simulink model "TC_track"  (R2026a)
settings: Solver=FixedStepDiscrete  StopTime=timeMax  FixedStep=Ts_plant
InitFcn:
  | TC_paramsOnly = true;
  | run('params_track.m');
  | clear TC_paramsOnly
values from neighbouring files (symbols this model uses):
  aeroFrontFraction = 0.50    (= 0.5)    [TC_parameters.m]    (also in params.m; params_track.m)
  CDA = 1.20    (= 1.2)    [TC_parameters.m]    (also in params.m; params_track.m)
  cg_f = W * rearWeightFraction    (= 0.765175)    [TC_parameters.m]    (also in params.m; params_track.m)
  cg_r = W * frontWeightFraction    (= 0.765175)    [TC_parameters.m]    (also in params.m; params_track.m)
  CLA = 4.40    (= 4.4)    [TC_parameters.m]    (also in params.m; params_track.m)
  Cmax = 0    [TC_parameters.m]    (also in params.m = 5.375; params_track.m = 5.375)
  Cmin = -Max_Motor_Torque    (= -21.5)    [TC_parameters.m]    (also in params.m; params_track.m)
  Course_Length = Track_Length    [params_track.m]
  Drive_Train = 0.85    [TC_parameters.m]    (also in params.m = 0.92; params_track.m = 0.92)
  Driver_Brake_Band = 1.0    (= 1)    [params_track.m]
  Driver_Brake_Max_Decel = 1.5*gravity    (= 14.709975)    [params_track.m]
  Driver_Lift_Band = 0.5    [params_track.m]
  Driver_Line_Recovery_Hz = 0.3    [params_track.m]
  Driver_Preview_Time = 0.3    [params_track.m]
  Driver_Speed_Target = speedCap*ones(size(Track_Curvature))    [params_track.m]
  fd = 12.5    [TC_parameters.m]    (also in params.m; params_track.m)
  Feedforward_FallRate_FL = 2000    [params.m]    (also in params_track.m)
  Feedforward_FallRate_FR = 2000    [params.m]    (also in params_track.m)
  Feedforward_FallRate_RL = 2000    [params.m]    (also in params_track.m)
  Feedforward_FallRate_RR = 2000    [params.m]    (also in params_track.m)
  Feedforward_Filter_Alpha = 1 - exp(-2*pi*Feedforward_Filter_Hz*Ts)    [params.m]    (also in params_track.m)
  Feedforward_InitialState_FL = muFz_front_launch / Feedforward_Filter_Alpha    [params.m]    (also in params_track.m)
  Feedforward_InitialState_FR = Feedforward_InitialState_FL    [params.m]    (also in params_track.m)
  Feedforward_InitialState_RL = muFz_rear_launch / Feedforward_Filter_Alpha    [params.m]    (also in params_track.m)
  Feedforward_InitialState_RR = Feedforward_InitialState_RL    [params.m]    (also in params_track.m)
  Feedforward_Launch_FL = min(Max_Motor_Torque, Kff_FL*r/(fd*Drive_Train) *      muFz_front_launch*targetForceShape(Slip_Target_FL))    [params.m]    (also in params_track.m)
  Feedforward_Launch_FR = min(Max_Motor_Torque, Kff_FR*r/(fd*Drive_Train) *      muFz_front_launch*targetForceShape(Slip_Target_FR))    [params.m]    (also in params_track.m)
  Feedforward_Launch_RL = min(Max_Motor_Torque, Kff_RL*r/(fd*Drive_Train) *      muFz_rear_launch*targetForceShape(Slip_Target_RL))    [params.m]    (also in params_track.m)
  Feedforward_Launch_RR = min(Max_Motor_Torque, Kff_RR*r/(fd*Drive_Train) *      muFz_rear_launch*targetForceShape(Slip_Target_RR))    [params.m]    (also in params_track.m)
  Feedforward_RiseRate_FL = 800    [params.m]    (also in params_track.m)
  Feedforward_RiseRate_FR = 800    [params.m]    (also in params_track.m)
  Feedforward_RiseRate_RL = 800    [params.m]    (also in params_track.m)
  Feedforward_RiseRate_RR = 800    [params.m]    (also in params_track.m)
  Fz_front_static = Mv * gravity * cg_r / W    (= 1387.6672151)    [TC_parameters.m]    (also in params.m; params_track.m)
  Fz_rear_static = Mv * gravity * cg_f / W    (= 1387.6672151)    [TC_parameters.m]    (also in params.m; params_track.m)
  Grip_Fact = 1.0    (= 1)    [TC_parameters.m]    (also in params.m = 0.6; params_track.m = 0.6)
  h_cg = 10.4 * in_to_m    (= 0.26416)    [TC_parameters.m]    (also in params.m; params_track.m)
  J_wheel_side = 0.45    [TC_parameters.m]    (also in params.m = 0.35; params_track.m = 0.35)
  Kaw_FL = Ki_FL / Kp_FL    (= 32)    [params.m]    (also in params_track.m)
  Kaw_FR = Ki_FR / Kp_FR    (= 32)    [params.m]    (also in params_track.m)
  Kaw_RL = Ki_RL / Kp_RL    (= 12)    [params.m]    (also in params_track.m)
  Kaw_RR = Ki_RR / Kp_RR    (= 12)    [params.m]    (also in params_track.m)
  Kd_FL = 0    [TC_parameters.m]    (also in params.m; params_track.m)
  Kd_FR = 0    [TC_parameters.m]    (also in params.m; params_track.m)
  Kd_RL = 0    [TC_parameters.m]    (also in params.m; params_track.m)
  Kd_RR = 0    [TC_parameters.m]    (also in params.m; params_track.m)
  Kff_FL = 0.9    [params.m]    (also in params_track.m)
  Kff_FR = 0.9    [params.m]    (also in params_track.m)
  Kff_RL = 0.9    [params.m]    (also in params_track.m)
  Kff_RR = 0.9    [params.m]    (also in params_track.m)
  Ki_FL = 180    [TC_parameters.m]    (also in params.m = 480; params_track.m = 480)
  Ki_FR = 180    [TC_parameters.m]    (also in params.m = 480; params_track.m = 480)
  Ki_RL = 180    [TC_parameters.m]    (also in params.m = 240; params_track.m = 240)
  Ki_RR = 180    [TC_parameters.m]    (also in params.m = 240; params_track.m = 240)
  Kp_FL = 32    [TC_parameters.m]    (also in params.m = 15; params_track.m = 15)
  Kp_FR = 32    [TC_parameters.m]    (also in params.m = 15; params_track.m = 15)
  Kp_RL = 32    [TC_parameters.m]    (also in params.m = 20; params_track.m = 20)
  Kp_RR = 32    [TC_parameters.m]    (also in params.m = 20; params_track.m = 20)
  Ktrack_FL = 50    [params.m]    (also in params_track.m)
  Ktrack_FR = 50    [params.m]    (also in params_track.m)
  Ktrack_RL = 50    [params.m]    (also in params_track.m)
  Ktrack_RR = 50    [params.m]    (also in params_track.m)
  Lateral_Mu_Ratio = 1.00    (= 1)    [params_track.m]
  Launch_Pedal_Initial = T_request_per_motor    (= 21.5)    [params.m]    (also in params_track.m)
  LLTD_Front = 0.50    (= 0.5)    [params_track.m]
  Max_Motor_Torque = 21.5    [TC_parameters.m]    (also in params.m; params_track.m)
  Max_Wheel_Omega = Max_Motor_RPM * 2*pi/60 / fd    (= 167.551608191)    [TC_parameters.m]    (also in params.m; params_track.m)
  maxTractivePower = 80e3    (= 80000)    [TC_parameters.m]    (also in params.m; params_track.m)
  motorInverterEfficiency = 1.00    (= 1)    [params.m]    (also in params_track.m)
  Mv = vehicleMassNoDriver + driverMass    (= 283.00535149)    [TC_parameters.m]    (also in params.m; params_track.m)
  Pacejka_B = 10.400    (= 10.4)    [TC_parameters.m]    (also in params.m; params_track.m)
  Pacejka_C = -1.580    (= -1.58)    [TC_parameters.m]    (also in params.m; params_track.m)
  Pacejka_D1 = -3.020    (= -3.02)    [TC_parameters.m]    (also in params.m; params_track.m)
  Pacejka_D2 = 0.800    (= 0.8)    [TC_parameters.m]    (also in params.m; params_track.m)
  r = 0.5 * 16.0 * in_to_m    (= 0.2032)    [TC_parameters.m]    (also in params.m; params_track.m; slip_estimator.m = ay / vref0)
  rho = 1.225    [TC_parameters.m]    (also in params.m; params_track.m)
  Slip_Filter_Alpha = 1 - exp(-2*pi*Slip_Filter_Hz*Ts)    [params.m]    (also in params_track.m)
  Slip_Target_FL = 0.12    [TC_parameters.m]    (also in params.m; params_track.m)
  Slip_Target_FR = 0.12    [TC_parameters.m]    (also in params.m; params_track.m)
  Slip_Target_RL = 0.12    [TC_parameters.m]    (also in params.m = 0.145; params_track.m = 0.145)
  Slip_Target_RR = 0.12    [TC_parameters.m]    (also in params.m = 0.145; params_track.m = 0.145)
  slipSpeedFloor = 0.50    (= 0.5)    [TC_parameters.m]    (also in params.m; params_track.m)
  Speed_Limit_Taper_Omega = Speed_Limit_Taper_RPM * 2*pi/60 / fd    (= 4.18879020479)    [params.m]    (also in params_track.m)
  Surface_Breakpoints = unique(surfaceBreaks)    [params_track.m]
  Surface_Grip_Table = Grip_Fact*ones(2, numel(Surface_Breakpoints))    [params_track.m]
  tau_motor = 0.03    [TC_parameters.m]    (also in params.m = 0.005; params_track.m = 0.005)
  Track_Breakpoints = double(misTrack.s_m(:))    [params_track.m]
  Track_Curvature = atGpsDistance(misTrack.curvature_1pm)    [params_track.m]
  trackFront = 49.0 * in_to_m    (= 1.2446)    [TC_parameters.m]    (also in params.m; params_track.m)
  trackRear = 49.0 * in_to_m    (= 1.2446)    [TC_parameters.m]    (also in params.m; params_track.m)
  Ts = 0.002    [TC_parameters.m]    (also in params.m; params_track.m)
  Ts_plant = 0.0001    [params.m]    (also in params_track.m)
  W = 60.25 * in_to_m    (= 1.53035)    [TC_parameters.m]    (also in params.m; params_track.m)
  Wheel_Lateral_Position = [trackFront/2; -trackFront/2;      trackRear/2; -trackRear/2]    [params_track.m]
  Wheel_Longitudinal_Position = [cg_f; cg_f; -cg_r; -cg_r]    [params_track.m]
  Wheel_Side = [1; 2; 1; 2]    [params_track.m]
undefined symbols (not defined in the file or in its folder): DiscIntNeverNeededParam
libraries: slpidlib x4
(part 1 of 2)
settings Model: Creator=jacks  LastModifiedBy=jacks

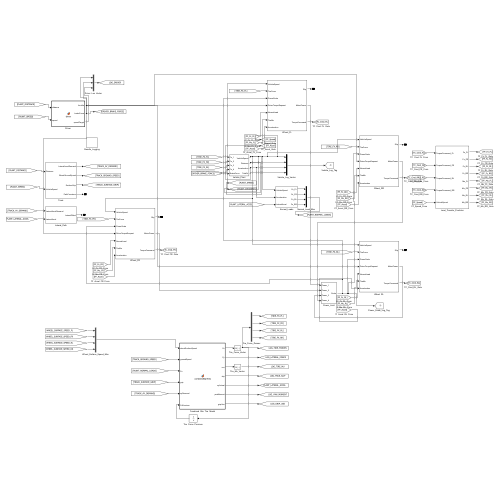
[thumbnail: Simulink's stored preview of the top-level diagram]
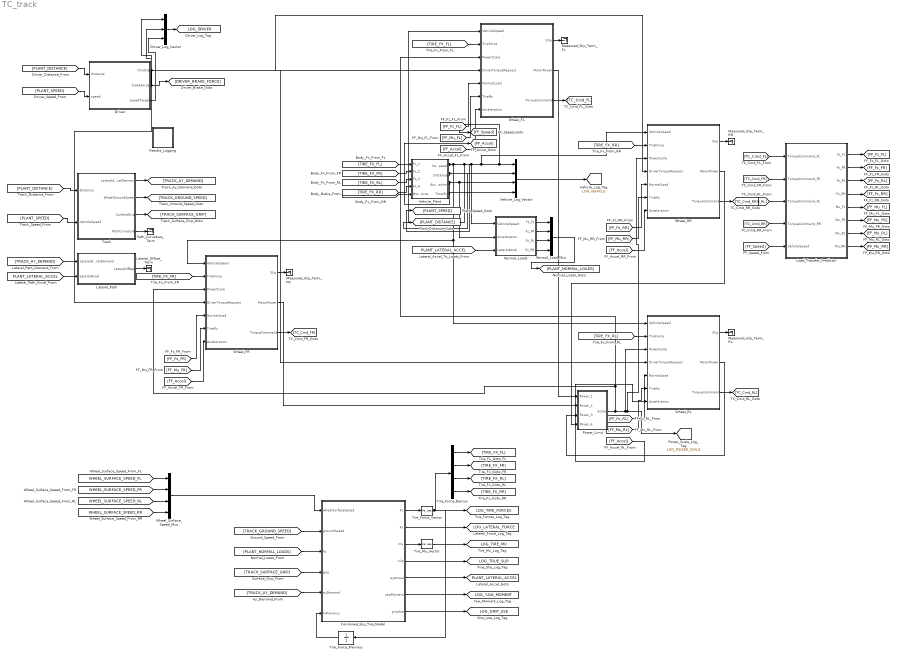
== system TC_track ==
  Combined_Slip_Tire_Model : MATLAB Function  TreatAsAtomicUnit=on
  Driver : MATLAB Function  TreatAsAtomicUnit=on
  Driver_Log_Vector : Mux  Inputs=3
  Lateral_Offset_Term : Terminator
  Lateral_Path : Subsystem  Description=Offset of the car left of the line. While the tires are short of the lateral acceleration the line needs, the car drifts by the difference; otherwise the driver steers back at Driver_Line_Recovery_Hz.
  Load_Transfer_Predictor : Subsystem
  Measured_Slip_Term_FL : Terminator
  Measured_Slip_Term_FR : Terminator
  Measured_Slip_Term_RL : Terminator
  Measured_Slip_Term_RR : Terminator
  Normal_Load_Mux : Mux
  Normal_Loads : Subsystem
  Path_Curvature_Term : Terminator
  Power_Limit : Subsystem
  Results_Logging : Subsystem
  Tire_Force_Demux : Demux
  Tire_Force_Previous : UnitDelay  InitialCondition=zeros(4,1)  SampleTime=Ts_plant
  Tire_Force_Vector : Reshape
  Tire_Mu_Vector : Reshape
  Track : Subsystem  Description=Track: path curvature, lateral-acceleration demand, per-wheel ground speeds, and per-wheel surface grip along the course.
  Vehicle_Log_Vector : Mux
  Vehicle_Plant : Subsystem
  Wheel_FL : Subsystem
  Wheel_FR : Subsystem
  Wheel_RL : Subsystem
  Wheel_RR : Subsystem
  Wheel_Surface_Speed_Mux : Mux
  tag scope: LOG_DRIVER=global, LOG_GRIP_USE=global, LOG_LATERAL_FORCE=global, LOG_POWER_SCALE=global, LOG_TIRE_FORCES=global, LOG_TIRE_MU=global, LOG_TRUE_SLIP=global, LOG_VEHICLE=global, LOG_YAW_MOMENT=global, PLANT_LATERAL_ACCEL=global
  wires:
  Power_Limit/1(Scale) -> [LOG_POWER_SCALE], Wheel_RR/3(PowerScale), Wheel_RL/3(PowerScale), Wheel_FR/3(PowerScale), Wheel_FL/3(PowerScale)
  Wheel_RR/2(MotorPower) -> Power_Limit/4(Power_4)
  Vehicle_Plant/1(VehicleSpeed) -> [FF_Speed], Vehicle_Log_Vector/1, Wheel_RR/1(VehicleSpeed), Normal_Loads/1(VehicleSpeed), Wheel_FL/1(VehicleSpeed), Wheel_RL/1(VehicleSpeed), Wheel_FR/1(VehicleSpeed), [PLANT_SPEED]
  Vehicle_Plant/3(Acceleration) -> Normal_Loads/2(Acceleration), Vehicle_Log_Vector/3, [FF_Accel]
  Vehicle_Plant/4(TotalFx) -> Vehicle_Log_Vector/4
  Vehicle_Plant/2(Distance) -> Vehicle_Log_Vector/2, [PLANT_DISTANCE]
  Wheel_RL/2(MotorPower) -> Power_Limit/3(Power_3)
  Wheel_FR/2(MotorPower) -> Power_Limit/2(Power_2)
  Wheel_FL/2(MotorPower) -> Power_Limit/1(Power_1)
  Vehicle_Log_Vector/1 -> [LOG_VEHICLE]
  [FF_Fz_FL] -> Wheel_FL/5(NormalLoad)
  [FF_Mu_FL] -> Wheel_FL/6(TireMu)
  [FF_Accel] -> Wheel_FL/7(Acceleration)
  [FF_Fz_FR] -> Wheel_FR/5(NormalLoad)
  [FF_Mu_FR] -> Wheel_FR/6(TireMu)
  [FF_Accel] -> Wheel_FR/7(Acceleration)
  [FF_Fz_RL] -> Wheel_RL/5(NormalLoad)
  [FF_Mu_RL] -> Wheel_RL/6(TireMu)
  [FF_Accel] -> Wheel_RL/7(Acceleration)
  [FF_Fz_RR] -> Wheel_RR/5(NormalLoad)
  [FF_Mu_RR] -> Wheel_RR/6(TireMu)
  [FF_Accel] -> Wheel_RR/7(Acceleration)
  Wheel_FL/3(TorqueCommand) -> [TC_Cmd_FL]
  [TC_Cmd_FL] -> Load_Transfer_Predictor/1(TorqueCommand_FL)
  Load_Transfer_Predictor/1(Fz_FL) -> [FF_Fz_FL]
  Load_Transfer_Predictor/5(Mu_FL) -> [FF_Mu_FL]
  Wheel_FR/3(TorqueCommand) -> [TC_Cmd_FR]
  [TC_Cmd_FR] -> Load_Transfer_Predictor/2(TorqueCommand_FR)
  Load_Transfer_Predictor/2(Fz_FR) -> [FF_Fz_FR]
  Load_Transfer_Predictor/6(Mu_FR) -> [FF_Mu_FR]
  Wheel_RL/3(TorqueCommand) -> [TC_Cmd_RL]
  [TC_Cmd_RL] -> Load_Transfer_Predictor/3(TorqueCommand_RL)
  Load_Transfer_Predictor/3(Fz_RL) -> [FF_Fz_RL]
  Load_Transfer_Predictor/7(Mu_RL) -> [FF_Mu_RL]
  Wheel_RR/3(TorqueCommand) -> [TC_Cmd_RR]
  [TC_Cmd_RR] -> Load_Transfer_Predictor/4(TorqueCommand_RR)
  Load_Transfer_Predictor/4(Fz_RR) -> [FF_Fz_RR]
  Load_Transfer_Predictor/8(Mu_RR) -> [FF_Mu_RR]
  [FF_Speed] -> Load_Transfer_Predictor/5(VehicleSpeed)
  Wheel_FL/1(Slip) -> Measured_Slip_Term_FL/1
  Wheel_FR/1(Slip) -> Measured_Slip_Term_FR/1
  Wheel_RL/1(Slip) -> Measured_Slip_Term_RL/1
  Wheel_RR/1(Slip) -> Measured_Slip_Term_RR/1
  [PLANT_DISTANCE] -> Track/1(Distance)
  [PLANT_SPEED] -> Track/2(VehicleSpeed)
  Track/1(LateralAccelDemand) -> [TRACK_AY_DEMAND]
  Track/2(WheelGroundSpeed) -> [TRACK_GROUND_SPEED]
  Track/3(SurfaceGrip) -> [TRACK_SURFACE_GRIP]
  Track/4(PathCurvature) -> Path_Curvature_Term/1
  Normal_Loads/1(Fz_FL) -> Normal_Load_Mux/1
  Normal_Loads/2(Fz_FR) -> Normal_Load_Mux/2
  Normal_Loads/3(Fz_RL) -> Normal_Load_Mux/3
  Normal_Loads/4(Fz_RR) -> Normal_Load_Mux/4
  Normal_Load_Mux/1 -> [PLANT_NORMAL_LOADS]
  [PLANT_LATERAL_ACCEL] -> Normal_Loads/3(LateralAccel)
  [WHEEL_SURFACE_SPEED_FL] -> Wheel_Surface_Speed_Mux/1
  [WHEEL_SURFACE_SPEED_FR] -> Wheel_Surface_Speed_Mux/2
  [WHEEL_SURFACE_SPEED_RL] -> Wheel_Surface_Speed_Mux/3
  [WHEEL_SURFACE_SPEED_RR] -> Wheel_Surface_Speed_Mux/4
  Wheel_Surface_Speed_Mux/1 -> Combined_Slip_Tire_Model/1(wheelSurfaceSpeed)
  [TRACK_GROUND_SPEED] -> Combined_Slip_Tire_Model/2(groundSpeed)
  [PLANT_NORMAL_LOADS] -> Combined_Slip_Tire_Model/3(Fz)
  [TRACK_SURFACE_GRIP] -> Combined_Slip_Tire_Model/4(grip)
  [TRACK_AY_DEMAND] -> Combined_Slip_Tire_Model/5(ayDemand)
  Combined_Slip_Tire_Model/1(Fx) -> Tire_Force_Vector/1
  Tire_Force_Vector/1 -> Tire_Force_Demux/1, [LOG_TIRE_FORCES], Tire_Force_Previous/1
  Tire_Force_Previous/1 -> Combined_Slip_Tire_Model/6(FxPrevious)
  Tire_Force_Demux/1 -> [TIRE_FX_FL]
  Tire_Force_Demux/2 -> [TIRE_FX_FR]
  Tire_Force_Demux/3 -> [TIRE_FX_RL]
  Tire_Force_Demux/4 -> [TIRE_FX_RR]
  [TIRE_FX_FL] -> Wheel_FL/2(TireForce)
  [TIRE_FX_FL] -> Vehicle_Plant/1(Fx_1)
  [TIRE_FX_FR] -> Wheel_FR/2(TireForce)
  [TIRE_FX_FR] -> Vehicle_Plant/2(Fx_2)
  [TIRE_FX_RL] -> Wheel_RL/2(TireForce)
  [TIRE_FX_RL] -> Vehicle_Plant/3(Fx_3)
  [TIRE_FX_RR] -> Wheel_RR/2(TireForce)
  [TIRE_FX_RR] -> Vehicle_Plant/4(Fx_4)
  Combined_Slip_Tire_Model/3(mu) -> Tire_Mu_Vector/1
  Tire_Mu_Vector/1 -> [LOG_TIRE_MU]
  [TRACK_AY_DEMAND] -> Lateral_Path/1(LateralAccelDemand)
  [PLANT_LATERAL_ACCEL] -> Lateral_Path/2(LateralAccel)
  Lateral_Path/1(LateralOffset) -> Lateral_Offset_Term/1
  Combined_Slip_Tire_Model/2(Fy) -> [LOG_LATERAL_FORCE]
  Combined_Slip_Tire_Model/4(slip) -> [LOG_TRUE_SLIP]
  Combined_Slip_Tire_Model/5(ayActual) -> [PLANT_LATERAL_ACCEL]
  Combined_Slip_Tire_Model/6(yawMoment) -> [LOG_YAW_MOMENT]
  Combined_Slip_Tire_Model/7(gripUse) -> [LOG_GRIP_USE]
  Driver/1(throttle) -> Wheel_RR/4(DriverTorqueRequest), Wheel_FL/4(DriverTorqueRequest), Wheel_FR/4(DriverTorqueRequest), Wheel_RL/4(DriverTorqueRequest), Driver_Log_Vector/1
  [PLANT_DISTANCE] -> Driver/1(distance)
  [PLANT_SPEED] -> Driver/2(speed)
  Driver/2(brakeForce) -> [DRIVER_BRAKE_FORCE], Driver_Log_Vector/2
  Driver/3(speedTarget) -> Driver_Log_Vector/3
  Driver_Log_Vector/1 -> [LOG_DRIVER]
  [DRIVER_BRAKE_FORCE] -> Vehicle_Plant/5(BrakeForce)

== system TC_track/Lateral_Path ==
  LateralAccelDemand : Inport
  LateralAccel : Inport  Port=2
  Achieved_Magnitude : Abs
  Demand_Magnitude : Abs
  Grip_Shortfall : Sum  Inputs=+-
  LateralOffsetLog : ToWorkspace  VariableName=lateralOffset  SaveFormat=Timeseries  SampleTime=-1
  Lateral_Accel_Error : Sum  Inputs=+-
  Lateral_Offset : DiscreteIntegrator  SampleTime=Ts_plant  ICPrevOutput=DiscIntNeverNeededParam  ICPrevScaledInput=DiscIntNeverNeededParam
  Lateral_Velocity : DiscreteIntegrator  SampleTime=Ts_plant  ICPrevOutput=DiscIntNeverNeededParam  ICPrevScaledInput=DiscIntNeverNeededParam
  Short_Of_Grip : Switch  Criteria=u2 > Threshold  Threshold=0.01
  Steer_Back_Accel : Sum
  Steer_Back_Damping : Gain  Gain=-4*pi*Driver_Line_Recovery_Hz
  Steer_Back_Stiffness : Gain  Gain=-(2*pi*Driver_Line_Recovery_Hz)^2
  LateralOffset : Outport
  wires:
  Demand_Magnitude/1 -> Grip_Shortfall/1
  Lateral_Accel_Error/1 -> Short_Of_Grip/1
  LateralAccel/1 -> Lateral_Accel_Error/1, Achieved_Magnitude/1
  LateralAccelDemand/1 -> Lateral_Accel_Error/2, Demand_Magnitude/1
  Achieved_Magnitude/1 -> Grip_Shortfall/2
  Grip_Shortfall/1 -> Short_Of_Grip/2
  Steer_Back_Damping/1 -> Steer_Back_Accel/1
  Steer_Back_Stiffness/1 -> Steer_Back_Accel/2
  Lateral_Velocity/1 -> Steer_Back_Damping/1, Lateral_Offset/1
  Steer_Back_Accel/1 -> Short_Of_Grip/3
  Short_Of_Grip/1 -> Lateral_Velocity/1
  Lateral_Offset/1 -> Steer_Back_Stiffness/1, LateralOffset/1, LateralOffsetLog/1

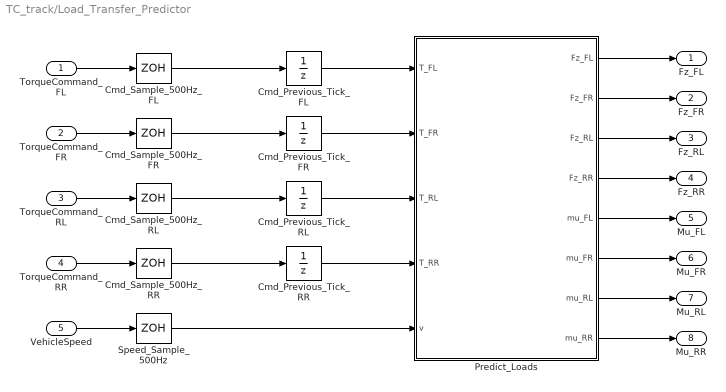
== system TC_track/Load_Transfer_Predictor ==
  TorqueCommand_FL : Inport
  TorqueCommand_FR : Inport  Port=2
  TorqueCommand_RL : Inport  Port=3
  TorqueCommand_RR : Inport  Port=4
  VehicleSpeed : Inport  Port=5
  Cmd_Previous_Tick_FL : UnitDelay  InitialCondition=Feedforward_Launch_FL  SampleTime=Ts
  Cmd_Previous_Tick_FR : UnitDelay  InitialCondition=Feedforward_Launch_FR  SampleTime=Ts
  Cmd_Previous_Tick_RL : UnitDelay  InitialCondition=Feedforward_Launch_RL  SampleTime=Ts
  Cmd_Previous_Tick_RR : UnitDelay  InitialCondition=Feedforward_Launch_RR  SampleTime=Ts
  Cmd_Sample_500Hz_FL : ZeroOrderHold  SampleTime=Ts
  Cmd_Sample_500Hz_FR : ZeroOrderHold  SampleTime=Ts
  Cmd_Sample_500Hz_RL : ZeroOrderHold  SampleTime=Ts
  Cmd_Sample_500Hz_RR : ZeroOrderHold  SampleTime=Ts
  Predict_Loads : MATLAB Function  TreatAsAtomicUnit=on
  Speed_Sample_500Hz : ZeroOrderHold  SampleTime=Ts
  Fz_FL : Outport
  Fz_FR : Outport  Port=2
  Fz_RL : Outport  Port=3
  Fz_RR : Outport  Port=4
  Mu_FL : Outport  Port=5
  Mu_FR : Outport  Port=6
  Mu_RL : Outport  Port=7
  Mu_RR : Outport  Port=8
  wires:
  TorqueCommand_FL/1 -> Cmd_Sample_500Hz_FL/1
  Cmd_Sample_500Hz_FL/1 -> Cmd_Previous_Tick_FL/1
  Cmd_Previous_Tick_FL/1 -> Predict_Loads/1(T_FL)
  TorqueCommand_FR/1 -> Cmd_Sample_500Hz_FR/1
  Cmd_Sample_500Hz_FR/1 -> Cmd_Previous_Tick_FR/1
  Cmd_Previous_Tick_FR/1 -> Predict_Loads/2(T_FR)
  TorqueCommand_RL/1 -> Cmd_Sample_500Hz_RL/1
  Cmd_Sample_500Hz_RL/1 -> Cmd_Previous_Tick_RL/1
  Cmd_Previous_Tick_RL/1 -> Predict_Loads/3(T_RL)
  TorqueCommand_RR/1 -> Cmd_Sample_500Hz_RR/1
  Cmd_Sample_500Hz_RR/1 -> Cmd_Previous_Tick_RR/1
  Cmd_Previous_Tick_RR/1 -> Predict_Loads/4(T_RR)
  VehicleSpeed/1 -> Speed_Sample_500Hz/1
  Speed_Sample_500Hz/1 -> Predict_Loads/5(v)
  Predict_Loads/1(Fz_FL) -> Fz_FL/1
  Predict_Loads/2(Fz_FR) -> Fz_FR/1
  Predict_Loads/3(Fz_RL) -> Fz_RL/1
  Predict_Loads/4(Fz_RR) -> Fz_RR/1
  Predict_Loads/5(mu_FL) -> Mu_FL/1
  Predict_Loads/6(mu_FR) -> Mu_FR/1
  Predict_Loads/7(mu_RL) -> Mu_RL/1
  Predict_Loads/8(mu_RR) -> Mu_RR/1

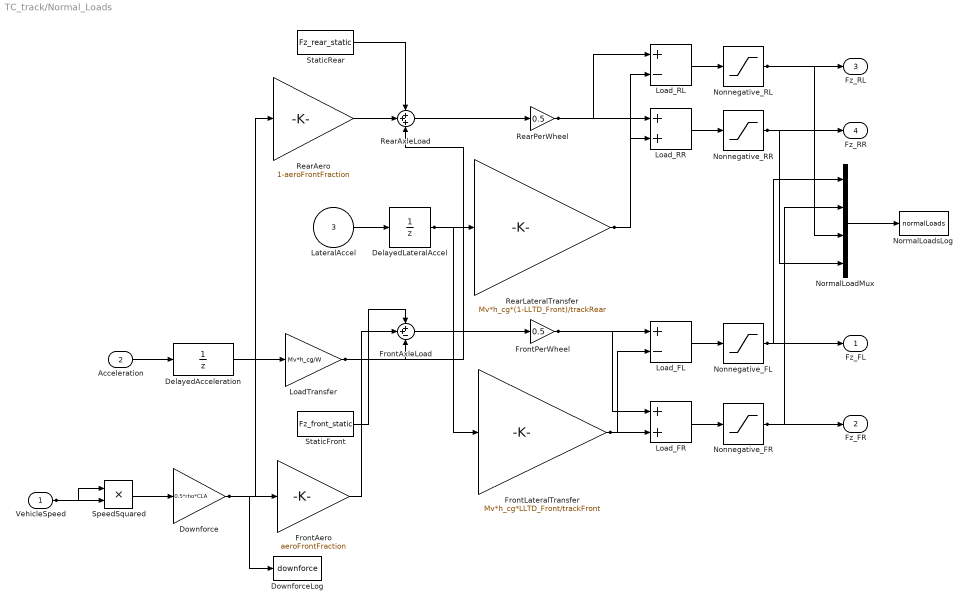
== system TC_track/Normal_Loads ==
  VehicleSpeed : Inport
  Acceleration : Inport  Port=2
  LateralAccel : Inport  Port=3
  DelayedAcceleration : UnitDelay  SampleTime=Ts_plant
  DelayedLateralAccel : UnitDelay  SampleTime=Ts_plant
  Downforce : Gain  Gain=0.5*rho*CLA
  DownforceLog : ToWorkspace  VariableName=downforce  SaveFormat=Timeseries  SampleTime=-1
  FrontAero : Gain  Gain=aeroFrontFraction
  FrontAxleLoad : Sum  Inputs=++-
  FrontLateralTransfer : Gain  Gain=Mv*h_cg*LLTD_Front/trackFront
  FrontPerWheel : Gain  Gain=0.5
  LoadTransfer : Gain  Gain=Mv*h_cg/W
  Load_FL : Sum  Inputs=+-
  Load_FR : Sum
  Load_RL : Sum  Inputs=+-
  Load_RR : Sum
  Nonnegative_FL : Saturate  UpperLimit=inf  LowerLimit=0
  Nonnegative_FR : Saturate  UpperLimit=inf  LowerLimit=0
  Nonnegative_RL : Saturate  UpperLimit=inf  LowerLimit=0
  Nonnegative_RR : Saturate  UpperLimit=inf  LowerLimit=0
  NormalLoadMux : Mux
  NormalLoadsLog : ToWorkspace  VariableName=normalLoads  SaveFormat=Timeseries  SampleTime=-1
  RearAero : Gain  Gain=1-aeroFrontFraction
  RearAxleLoad : Sum  Inputs=+++
  RearLateralTransfer : Gain  Gain=Mv*h_cg*(1-LLTD_Front)/trackRear
  RearPerWheel : Gain  Gain=0.5
  SpeedSquared : Product  Inputs=**
  StaticFront : Constant  Value=Fz_front_static
  StaticRear : Constant  Value=Fz_rear_static
  Fz_FL : Outport
  Fz_FR : Outport  Port=2
  Fz_RL : Outport  Port=3
  Fz_RR : Outport  Port=4
  wires:
  FrontAxleLoad/1 -> FrontPerWheel/1
  VehicleSpeed/1 -> SpeedSquared/1, SpeedSquared/2
  Downforce/1 -> DownforceLog/1, FrontAero/1, RearAero/1
  DelayedAcceleration/1 -> LoadTransfer/1
  Acceleration/1 -> DelayedAcceleration/1
  StaticFront/1 -> FrontAxleLoad/1
  LateralAccel/1 -> DelayedLateralAccel/1
  DelayedLateralAccel/1 -> FrontLateralTransfer/1, RearLateralTransfer/1
  RearAero/1 -> RearAxleLoad/2
  SpeedSquared/1 -> Downforce/1
  StaticRear/1 -> RearAxleLoad/1
  LoadTransfer/1 -> RearAxleLoad/3, FrontAxleLoad/3
  FrontAero/1 -> FrontAxleLoad/2
  RearAxleLoad/1 -> RearPerWheel/1
  NormalLoadMux/1 -> NormalLoadsLog/1
  RearPerWheel/1 -> Load_RL/1, Load_RR/1
  Load_RR/1 -> Nonnegative_RR/1
  RearLateralTransfer/1 -> Load_RL/2, Load_RR/2
  FrontPerWheel/1 -> Load_FR/1, Load_FL/1
  Load_FR/1 -> Nonnegative_FR/1
  FrontLateralTransfer/1 -> Load_FL/2, Load_FR/2
  Load_RL/1 -> Nonnegative_RL/1
  Load_FL/1 -> Nonnegative_FL/1
  Nonnegative_RL/1 -> NormalLoadMux/3, Fz_RL/1
  Nonnegative_RR/1 -> NormalLoadMux/4, Fz_RR/1
  Nonnegative_FL/1 -> NormalLoadMux/1, Fz_FL/1
  Nonnegative_FR/1 -> NormalLoadMux/2, Fz_FR/1

== system TC_track/Power_Limit ==
  Power_1 : Inport
  Power_2 : Inport  Port=2
  Power_3 : Inport  Port=3
  Power_4 : Inport  Port=4
  LimitRatio : Product  Inputs=*/
  PowerFloor : Constant
  PowerLimit : Constant  Value=maxTractivePower
  PowerScale : MinMax  Inputs=2
  Power_1_Sample_500Hz : ZeroOrderHold  SampleTime=Ts
  Power_2_Sample_500Hz : ZeroOrderHold  SampleTime=Ts
  Power_3_Sample_500Hz : ZeroOrderHold  SampleTime=Ts
  Power_4_Sample_500Hz : ZeroOrderHold  SampleTime=Ts
  Power_Command_Delay_2ms : UnitDelay  InitialCondition=1  SampleTime=Ts
  SafePower : MinMax  Function=max  Inputs=2
  TotalPower : Sum  Inputs=++++
  Unity : Constant
  Scale : Outport
  wires:
  Power_Command_Delay_2ms/1 -> Scale/1
  Power_4_Sample_500Hz/1 -> TotalPower/4
  Power_3_Sample_500Hz/1 -> TotalPower/3
  Power_2_Sample_500Hz/1 -> TotalPower/2
  Power_1_Sample_500Hz/1 -> TotalPower/1
  Power_2/1 -> Power_2_Sample_500Hz/1
  Power_3/1 -> Power_3_Sample_500Hz/1
  Power_4/1 -> Power_4_Sample_500Hz/1
  TotalPower/1 -> SafePower/1
  PowerFloor/1 -> SafePower/2
  PowerLimit/1 -> LimitRatio/1
  SafePower/1 -> LimitRatio/2
  LimitRatio/1 -> PowerScale/1
  Unity/1 -> PowerScale/2
  PowerScale/1 -> Power_Command_Delay_2ms/1
  Power_1/1 -> Power_1_Sample_500Hz/1

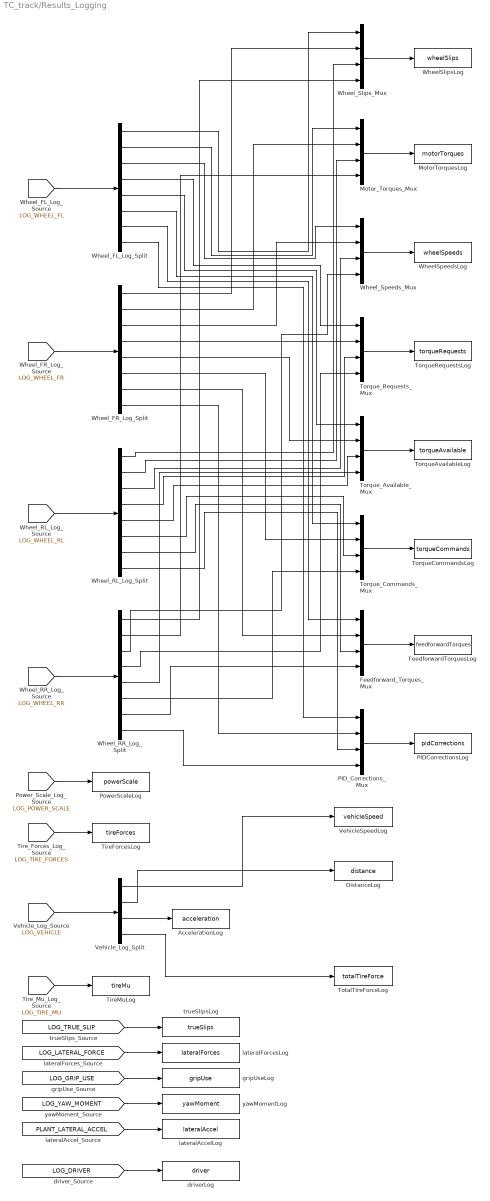
== system TC_track/Results_Logging ==
  AccelerationLog : ToWorkspace  VariableName=acceleration  SaveFormat=Timeseries  SampleTime=-1
  DistanceLog : ToWorkspace  VariableName=distance  SaveFormat=Timeseries  SampleTime=-1
  FeedforwardTorquesLog : ToWorkspace  VariableName=feedforwardTorques  SaveFormat=Timeseries  SampleTime=-1
  Feedforward_Torques_Mux : Mux
  MotorTorquesLog : ToWorkspace  VariableName=motorTorques  SaveFormat=Timeseries  SampleTime=-1
  Motor_Torques_Mux : Mux
  PIDCorrectionsLog : ToWorkspace  VariableName=pidCorrections  SaveFormat=Timeseries  SampleTime=-1
  PID_Corrections_Mux : Mux
  PowerScaleLog : ToWorkspace  VariableName=powerScale  SaveFormat=Timeseries  SampleTime=-1
  TireForcesLog : ToWorkspace  VariableName=tireForces  SaveFormat=Timeseries  SampleTime=-1
  TireMuLog : ToWorkspace  VariableName=tireMu  SaveFormat=Timeseries  SampleTime=-1
  TorqueAvailableLog : ToWorkspace  VariableName=torqueAvailable  SaveFormat=Timeseries  SampleTime=-1
  TorqueCommandsLog : ToWorkspace  VariableName=torqueCommands  SaveFormat=Timeseries  SampleTime=-1
  TorqueRequestsLog : ToWorkspace  VariableName=torqueRequests  SaveFormat=Timeseries  SampleTime=-1
  Torque_Available_Mux : Mux
  Torque_Commands_Mux : Mux
  Torque_Requests_Mux : Mux
  TotalTireForceLog : ToWorkspace  VariableName=totalTireForce  SaveFormat=Timeseries  SampleTime=-1
  VehicleSpeedLog : ToWorkspace  VariableName=vehicleSpeed  SaveFormat=Timeseries  SampleTime=-1
  Vehicle_Log_Split : Demux
  WheelSlipsLog : ToWorkspace  VariableName=wheelSlips  SaveFormat=Timeseries  SampleTime=-1
  WheelSpeedsLog : ToWorkspace  VariableName=wheelSpeeds  SaveFormat=Timeseries  SampleTime=-1
  Wheel_FL_Log_Split : Demux  Outputs=8
  Wheel_FR_Log_Split : Demux  Outputs=8
  Wheel_RL_Log_Split : Demux  Outputs=8
  Wheel_RR_Log_Split : Demux  Outputs=8
  Wheel_Slips_Mux : Mux
  Wheel_Speeds_Mux : Mux
  driverLog : ToWorkspace  VariableName=driver  SaveFormat=Timeseries  SampleTime=-1
  gripUseLog : ToWorkspace  VariableName=gripUse  SaveFormat=Timeseries  SampleTime=-1
  lateralAccelLog : ToWorkspace  VariableName=lateralAccel  SaveFormat=Timeseries  SampleTime=-1
  lateralForcesLog : ToWorkspace  VariableName=lateralForces  SaveFormat=Timeseries  SampleTime=-1
  trueSlipsLog : ToWorkspace  VariableName=trueSlips  SaveFormat=Timeseries  SampleTime=-1
  yawMomentLog : ToWorkspace  VariableName=yawMoment  SaveFormat=Timeseries  SampleTime=-1
  wires:
  [LOG_POWER_SCALE] -> PowerScaleLog/1
  Vehicle_Log_Split/4 -> TotalTireForceLog/1
  Vehicle_Log_Split/3 -> AccelerationLog/1
  Vehicle_Log_Split/2 -> DistanceLog/1
  Vehicle_Log_Split/1 -> VehicleSpeedLog/1
  [LOG_VEHICLE] -> Vehicle_Log_Split/1
  [LOG_TIRE_MU] -> TireMuLog/1
  [LOG_TIRE_FORCES] -> TireForcesLog/1
  PID_Corrections_Mux/1 -> PIDCorrectionsLog/1
  Wheel_RR_Log_Split/8 -> PID_Corrections_Mux/4
  Wheel_RL_Log_Split/8 -> PID_Corrections_Mux/3
  Wheel_FR_Log_Split/8 -> PID_Corrections_Mux/2
  Wheel_FL_Log_Split/8 -> PID_Corrections_Mux/1
  Feedforward_Torques_Mux/1 -> FeedforwardTorquesLog/1
  Wheel_RR_Log_Split/7 -> Feedforward_Torques_Mux/4
  Wheel_RL_Log_Split/7 -> Feedforward_Torques_Mux/3
  Wheel_FR_Log_Split/7 -> Feedforward_Torques_Mux/2
  Wheel_FL_Log_Split/7 -> Feedforward_Torques_Mux/1
  Torque_Commands_Mux/1 -> TorqueCommandsLog/1
  Wheel_RR_Log_Split/6 -> Torque_Commands_Mux/4
  Wheel_RL_Log_Split/6 -> Torque_Commands_Mux/3
  Wheel_FR_Log_Split/6 -> Torque_Commands_Mux/2
  Wheel_FL_Log_Split/6 -> Torque_Commands_Mux/1
  Torque_Available_Mux/1 -> TorqueAvailableLog/1
  Wheel_RR_Log_Split/5 -> Torque_Available_Mux/4
  Wheel_RL_Log_Split/5 -> Torque_Available_Mux/3
  Wheel_FR_Log_Split/5 -> Torque_Available_Mux/2
  Wheel_FL_Log_Split/5 -> Torque_Available_Mux/1
  Torque_Requests_Mux/1 -> TorqueRequestsLog/1
  Wheel_RR_Log_Split/4 -> Torque_Requests_Mux/4
  Wheel_RL_Log_Split/4 -> Torque_Requests_Mux/3
  Wheel_FR_Log_Split/4 -> Torque_Requests_Mux/2
  Wheel_FL_Log_Split/4 -> Torque_Requests_Mux/1
  Wheel_Speeds_Mux/1 -> WheelSpeedsLog/1
  Wheel_RR_Log_Split/3 -> Wheel_Speeds_Mux/4
  Wheel_RL_Log_Split/3 -> Wheel_Speeds_Mux/3
  Wheel_FR_Log_Split/3 -> Wheel_Speeds_Mux/2
  Wheel_FL_Log_Split/3 -> Wheel_Speeds_Mux/1
  Motor_Torques_Mux/1 -> MotorTorquesLog/1
  Wheel_RR_Log_Split/2 -> Motor_Torques_Mux/4
  Wheel_RL_Log_Split/2 -> Motor_Torques_Mux/3
  Wheel_FR_Log_Split/2 -> Motor_Torques_Mux/2
  Wheel_FL_Log_Split/2 -> Motor_Torques_Mux/1
  Wheel_Slips_Mux/1 -> WheelSlipsLog/1
  Wheel_RR_Log_Split/1 -> Wheel_Slips_Mux/4
  Wheel_RL_Log_Split/1 -> Wheel_Slips_Mux/3
  Wheel_FR_Log_Split/1 -> Wheel_Slips_Mux/2
  Wheel_FL_Log_Split/1 -> Wheel_Slips_Mux/1
  [LOG_WHEEL_RR] -> Wheel_RR_Log_Split/1
  [LOG_WHEEL_RL] -> Wheel_RL_Log_Split/1
  [LOG_WHEEL_FR] -> Wheel_FR_Log_Split/1
  [LOG_WHEEL_FL] -> Wheel_FL_Log_Split/1
  [LOG_TRUE_SLIP] -> trueSlipsLog/1
  [LOG_LATERAL_FORCE] -> lateralForcesLog/1
  [LOG_GRIP_USE] -> gripUseLog/1
  [LOG_YAW_MOMENT] -> yawMomentLog/1
  [PLANT_LATERAL_ACCEL] -> lateralAccelLog/1
  [LOG_DRIVER] -> driverLog/1

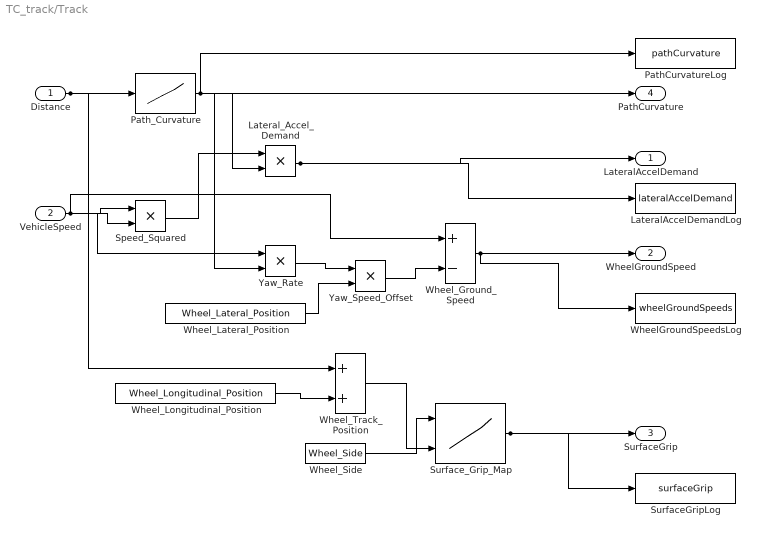
== system TC_track/Track ==
  Distance : Inport
  VehicleSpeed : Inport  Port=2
  LateralAccelDemandLog : ToWorkspace  VariableName=lateralAccelDemand  SaveFormat=Timeseries  SampleTime=-1
  Lateral_Accel_Demand : Product  Inputs=**
  PathCurvatureLog : ToWorkspace  VariableName=pathCurvature  SaveFormat=Timeseries  SampleTime=-1
  Path_Curvature : Lookup_n-D  NumberOfTableDimensions=1  BreakpointsForDimension1=Track_Breakpoints  Table=Track_Curvature  ExtrapMethod=Clip  InternalRulePriority=Speed  RndMeth=Simplest
  Speed_Squared : Product  Inputs=**
  SurfaceGripLog : ToWorkspace  VariableName=surfaceGrip  SaveFormat=Timeseries  SampleTime=-1
  Surface_Grip_Map : Lookup_n-D  BreakpointsForDimension1=[1 2]  BreakpointsForDimension2=Surface_Breakpoints  Table=Surface_Grip_Table  ExtrapMethod=Clip  InternalRulePriority=Speed  RndMeth=Simplest
      settings: InputPortMap=u0,u1
  WheelGroundSpeedsLog : ToWorkspace  VariableName=wheelGroundSpeeds  SaveFormat=Timeseries  SampleTime=-1
  Wheel_Ground_Speed : Sum  Inputs=+-
  Wheel_Lateral_Position : Constant  Value=Wheel_Lateral_Position
  Wheel_Longitudinal_Position : Constant  Value=Wheel_Longitudinal_Position
  Wheel_Side : Constant  Value=Wheel_Side
  Wheel_Track_Position : Sum
  Yaw_Rate : Product  Inputs=**
  Yaw_Speed_Offset : Product  Inputs=**
  LateralAccelDemand : Outport
  WheelGroundSpeed : Outport  Port=2
  SurfaceGrip : Outport  Port=3
  PathCurvature : Outport  Port=4
  wires:
  Distance/1 -> Path_Curvature/1, Wheel_Track_Position/1
  VehicleSpeed/1 -> Speed_Squared/1, Speed_Squared/2, Yaw_Rate/1, Wheel_Ground_Speed/1
  Speed_Squared/1 -> Lateral_Accel_Demand/1
  Path_Curvature/1 -> Lateral_Accel_Demand/2, Yaw_Rate/2, PathCurvature/1, PathCurvatureLog/1
  Yaw_Rate/1 -> Yaw_Speed_Offset/1
  Wheel_Lateral_Position/1 -> Yaw_Speed_Offset/2
  Yaw_Speed_Offset/1 -> Wheel_Ground_Speed/2
  Wheel_Longitudinal_Position/1 -> Wheel_Track_Position/2
  Wheel_Side/1 -> Surface_Grip_Map/1
  Wheel_Track_Position/1 -> Surface_Grip_Map/2
  Lateral_Accel_Demand/1 -> LateralAccelDemand/1, LateralAccelDemandLog/1
  Wheel_Ground_Speed/1 -> WheelGroundSpeed/1, WheelGroundSpeedsLog/1
  Surface_Grip_Map/1 -> SurfaceGrip/1, SurfaceGripLog/1

== system TC_track/Vehicle_Plant ==
  Fx_1 : Inport
  Fx_2 : Inport  Port=2
  Fx_3 : Inport  Port=3
  Fx_4 : Inport  Port=4
  BrakeForce : Inport  Port=5
  AeroDrag : Gain  Gain=0.5*rho*CDA
  AeroDragLog : ToWorkspace  VariableName=aeroDrag  SaveFormat=Timeseries  SampleTime=-1
  CourseEnd : Constant  Value=Course_Length
  DistanceState : DiscreteIntegrator  SampleTime=Ts_plant  ICPrevOutput=DiscIntNeverNeededParam  ICPrevScaledInput=DiscIntNeverNeededParam
  InvMass : Gain  Gain=1/Mv
  NetForce : Sum  Inputs=+--
  ReachedCourseEnd : RelationalOperator  OutDataTypeStr=boolean  RndMeth=Simplest  InputSameDT=off
  SpeedSquared : Product  Inputs=**
  StopAtCourseEnd : Stop
  TotalTireForce : Sum  Inputs=++++
  VehicleSpeedState : DiscreteIntegrator  SampleTime=Ts_plant  ICPrevOutput=DiscIntNeverNeededParam  ICPrevScaledInput=DiscIntNeverNeededParam
  VehicleSpeed : Outport
  Distance : Outport  Port=2
  Acceleration : Outport  Port=3
  TotalFx : Outport  Port=4
  wires:
  VehicleSpeedState/1 -> SpeedSquared/1, VehicleSpeed/1, DistanceState/1, SpeedSquared/2
  Fx_4/1 -> TotalTireForce/4
  Fx_3/1 -> TotalTireForce/3
  Fx_2/1 -> TotalTireForce/2
  DistanceState/1 -> ReachedCourseEnd/1, Distance/1
  Fx_1/1 -> TotalTireForce/1
  SpeedSquared/1 -> AeroDrag/1
  CourseEnd/1 -> ReachedCourseEnd/2
  ReachedCourseEnd/1 -> StopAtCourseEnd/1
  AeroDrag/1 -> NetForce/2, AeroDragLog/1
  TotalTireForce/1 -> NetForce/1, TotalFx/1
  BrakeForce/1 -> NetForce/3
  NetForce/1 -> InvMass/1
  InvMass/1 -> VehicleSpeedState/1, Acceleration/1

== system TC_track/Wheel_FL ==
  VehicleSpeed : Inport
  TireForce : Inport  Port=2
  PowerScale : Inport  Port=3
  DriverTorqueRequest : Inport  Port=4
  NormalLoad : Inport  Port=5
  TireMu : Inport  Port=6
  Acceleration : Inport  Port=7
  Logging_Vector : Mux  Inputs=8
  Motor_Wheel_Dynamics : Subsystem
  Slip_Estimator : Subsystem
  Traction_Controller_500Hz : Subsystem
  Slip : Outport
  MotorPower : Outport  Port=2
  TorqueCommand : Outport  Port=3
  tag scope: LOG_WHEEL_FL=global, WHEEL_SURFACE_SPEED_FL=global
  wires:
  TireForce/1 -> Motor_Wheel_Dynamics/3(TireForce)
  PowerScale/1 -> Motor_Wheel_Dynamics/2(PowerScale)
  Slip_Estimator/1(Slip) -> Logging_Vector/1, Slip/1, Traction_Controller_500Hz/1(Slip)
  Motor_Wheel_Dynamics/3(WheelSurfaceSpeed) -> Slip_Estimator/2(WheelSurfaceSpeed), Logging_Vector/3, [WHEEL_SURFACE_SPEED_FL]
  VehicleSpeed/1 -> Slip_Estimator/1(VehicleSpeed)
  DriverTorqueRequest/1 -> Traction_Controller_500Hz/2(DriverTorqueRequest)
  Traction_Controller_500Hz/1(TorqueRequested) -> Logging_Vector/4, Motor_Wheel_Dynamics/1(TorqueRequested)
  Motor_Wheel_Dynamics/1(MotorTorque) -> Logging_Vector/2
  Motor_Wheel_Dynamics/2(MotorPower) -> MotorPower/1
  Motor_Wheel_Dynamics/4(TorqueAvailable) -> Logging_Vector/5
  Motor_Wheel_Dynamics/5(TorqueCommand) -> Logging_Vector/6, TorqueCommand/1
  Traction_Controller_500Hz/2(FeedforwardTorque) -> Logging_Vector/7
  Traction_Controller_500Hz/3(PIDCorrection) -> Logging_Vector/8
  Logging_Vector/1 -> [LOG_WHEEL_FL]
  NormalLoad/1 -> Traction_Controller_500Hz/3(NormalLoad)
  TireMu/1 -> Traction_Controller_500Hz/4(TireMu)
  Acceleration/1 -> Traction_Controller_500Hz/5(Acceleration)

== system TC_track/Wheel_FR ==
  VehicleSpeed : Inport
  TireForce : Inport  Port=2
  PowerScale : Inport  Port=3
  DriverTorqueRequest : Inport  Port=4
  NormalLoad : Inport  Port=5
  TireMu : Inport  Port=6
  Acceleration : Inport  Port=7
  Logging_Vector : Mux  Inputs=8
  Motor_Wheel_Dynamics : Subsystem
  Slip_Estimator : Subsystem
  Traction_Controller_500Hz : Subsystem
  Slip : Outport
  MotorPower : Outport  Port=2
  TorqueCommand : Outport  Port=3
  tag scope: LOG_WHEEL_FR=global, WHEEL_SURFACE_SPEED_FR=global
  wires:
  VehicleSpeed/1 -> Slip_Estimator/1(VehicleSpeed)
  PowerScale/1 -> Motor_Wheel_Dynamics/2(PowerScale)
  TireForce/1 -> Motor_Wheel_Dynamics/3(TireForce)
  Motor_Wheel_Dynamics/3(WheelSurfaceSpeed) -> Logging_Vector/3, Slip_Estimator/2(WheelSurfaceSpeed), [WHEEL_SURFACE_SPEED_FR]
  Slip_Estimator/1(Slip) -> Logging_Vector/1, Slip/1, Traction_Controller_500Hz/1(Slip)
  DriverTorqueRequest/1 -> Traction_Controller_500Hz/2(DriverTorqueRequest)
  Traction_Controller_500Hz/1(TorqueRequested) -> Logging_Vector/4, Motor_Wheel_Dynamics/1(TorqueRequested)
  Motor_Wheel_Dynamics/1(MotorTorque) -> Logging_Vector/2
  Motor_Wheel_Dynamics/2(MotorPower) -> MotorPower/1
  Motor_Wheel_Dynamics/4(TorqueAvailable) -> Logging_Vector/5
  Motor_Wheel_Dynamics/5(TorqueCommand) -> Logging_Vector/6, TorqueCommand/1
  Traction_Controller_500Hz/2(FeedforwardTorque) -> Logging_Vector/7
  Traction_Controller_500Hz/3(PIDCorrection) -> Logging_Vector/8
  Logging_Vector/1 -> [LOG_WHEEL_FR]
  NormalLoad/1 -> Traction_Controller_500Hz/3(NormalLoad)
  TireMu/1 -> Traction_Controller_500Hz/4(TireMu)
  Acceleration/1 -> Traction_Controller_500Hz/5(Acceleration)

== system TC_track/Wheel_RL ==
  VehicleSpeed : Inport
  TireForce : Inport  Port=2
  PowerScale : Inport  Port=3
  DriverTorqueRequest : Inport  Port=4
  NormalLoad : Inport  Port=5
  TireMu : Inport  Port=6
  Acceleration : Inport  Port=7
  Logging_Vector : Mux  Inputs=8
  Motor_Wheel_Dynamics : Subsystem
  Slip_Estimator : Subsystem
  Traction_Controller_500Hz : Subsystem
  Slip : Outport
  MotorPower : Outport  Port=2
  TorqueCommand : Outport  Port=3
  tag scope: LOG_WHEEL_RL=global, WHEEL_SURFACE_SPEED_RL=global
  wires:
  VehicleSpeed/1 -> Slip_Estimator/1(VehicleSpeed)
  PowerScale/1 -> Motor_Wheel_Dynamics/2(PowerScale)
  TireForce/1 -> Motor_Wheel_Dynamics/3(TireForce)
  Motor_Wheel_Dynamics/3(WheelSurfaceSpeed) -> Logging_Vector/3, Slip_Estimator/2(WheelSurfaceSpeed), [WHEEL_SURFACE_SPEED_RL]
  Slip_Estimator/1(Slip) -> Logging_Vector/1, Slip/1, Traction_Controller_500Hz/1(Slip)
  DriverTorqueRequest/1 -> Traction_Controller_500Hz/2(DriverTorqueRequest)
  Traction_Controller_500Hz/1(TorqueRequested) -> Logging_Vector/4, Motor_Wheel_Dynamics/1(TorqueRequested)
  Motor_Wheel_Dynamics/1(MotorTorque) -> Logging_Vector/2
  Motor_Wheel_Dynamics/2(MotorPower) -> MotorPower/1
  Motor_Wheel_Dynamics/4(TorqueAvailable) -> Logging_Vector/5
  Motor_Wheel_Dynamics/5(TorqueCommand) -> Logging_Vector/6, TorqueCommand/1
  Traction_Controller_500Hz/2(FeedforwardTorque) -> Logging_Vector/7
  Traction_Controller_500Hz/3(PIDCorrection) -> Logging_Vector/8
  Logging_Vector/1 -> [LOG_WHEEL_RL]
  NormalLoad/1 -> Traction_Controller_500Hz/3(NormalLoad)
  TireMu/1 -> Traction_Controller_500Hz/4(TireMu)
  Acceleration/1 -> Traction_Controller_500Hz/5(Acceleration)

== system TC_track/Wheel_RR ==
  VehicleSpeed : Inport
  TireForce : Inport  Port=2
  PowerScale : Inport  Port=3
  DriverTorqueRequest : Inport  Port=4
  NormalLoad : Inport  Port=5
  TireMu : Inport  Port=6
  Acceleration : Inport  Port=7
  Logging_Vector : Mux  Inputs=8
  Motor_Wheel_Dynamics : Subsystem
  Slip_Estimator : Subsystem
  Traction_Controller_500Hz : Subsystem
  Slip : Outport
  MotorPower : Outport  Port=2
  TorqueCommand : Outport  Port=3
  tag scope: LOG_WHEEL_RR=global, WHEEL_SURFACE_SPEED_RR=global
  wires:
  VehicleSpeed/1 -> Slip_Estimator/1(VehicleSpeed)
  PowerScale/1 -> Motor_Wheel_Dynamics/2(PowerScale)
  TireForce/1 -> Motor_Wheel_Dynamics/3(TireForce)
  Motor_Wheel_Dynamics/3(WheelSurfaceSpeed) -> Logging_Vector/3, Slip_Estimator/2(WheelSurfaceSpeed), [WHEEL_SURFACE_SPEED_RR]
  Slip_Estimator/1(Slip) -> Logging_Vector/1, Slip/1, Traction_Controller_500Hz/1(Slip)
  DriverTorqueRequest/1 -> Traction_Controller_500Hz/2(DriverTorqueRequest)
  Traction_Controller_500Hz/1(TorqueRequested) -> Logging_Vector/4, Motor_Wheel_Dynamics/1(TorqueRequested)
  Motor_Wheel_Dynamics/1(MotorTorque) -> Logging_Vector/2
  Motor_Wheel_Dynamics/2(MotorPower) -> MotorPower/1
  Motor_Wheel_Dynamics/4(TorqueAvailable) -> Logging_Vector/5
  Motor_Wheel_Dynamics/5(TorqueCommand) -> Logging_Vector/6, TorqueCommand/1
  Traction_Controller_500Hz/2(FeedforwardTorque) -> Logging_Vector/7
  Traction_Controller_500Hz/3(PIDCorrection) -> Logging_Vector/8
  Logging_Vector/1 -> [LOG_WHEEL_RR]
  NormalLoad/1 -> Traction_Controller_500Hz/3(NormalLoad)
  TireMu/1 -> Traction_Controller_500Hz/4(TireMu)
  Acceleration/1 -> Traction_Controller_500Hz/5(Acceleration)

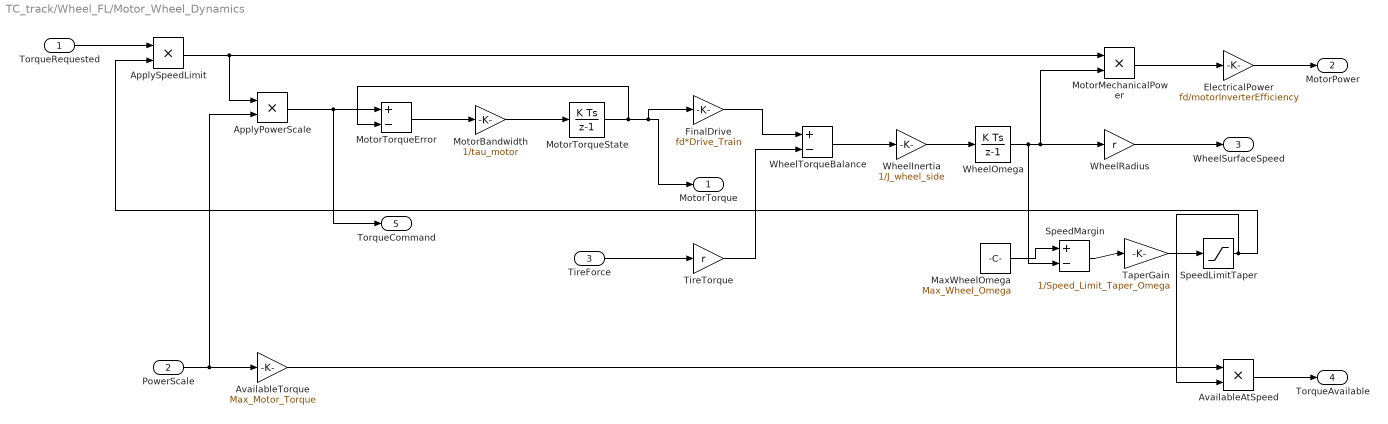
== system TC_track/Wheel_FL/Motor_Wheel_Dynamics ==
  TorqueRequested : Inport
  PowerScale : Inport  Port=2
  TireForce : Inport  Port=3
  ApplyPowerScale : Product
  ApplySpeedLimit : Product
  AvailableAtSpeed : Product
  AvailableTorque : Gain  Gain=Max_Motor_Torque
  ElectricalPower : Gain  Gain=fd/motorInverterEfficiency
  FinalDrive : Gain  Gain=fd*Drive_Train
  MaxWheelOmega : Constant  Value=Max_Wheel_Omega
  MotorBandwidth : Gain  Gain=1/tau_motor
  MotorMechanicalPower : Product
  MotorTorqueError : Sum  Inputs=+-
  MotorTorqueState : DiscreteIntegrator  SampleTime=Ts_plant  ICPrevOutput=DiscIntNeverNeededParam  ICPrevScaledInput=DiscIntNeverNeededParam
  SpeedLimitTaper : Saturate  UpperLimit=1  LowerLimit=0
  SpeedMargin : Sum  Inputs=+-
  TaperGain : Gain  Gain=1/Speed_Limit_Taper_Omega
  TireTorque : Gain  Gain=r
  WheelInertia : Gain  Gain=1/J_wheel_side
  WheelOmega : DiscreteIntegrator  SampleTime=Ts_plant  ICPrevOutput=DiscIntNeverNeededParam  ICPrevScaledInput=DiscIntNeverNeededParam
  WheelRadius : Gain  Gain=r
  WheelTorqueBalance : Sum  Inputs=+-
  MotorTorque : Outport
  MotorPower : Outport  Port=2
  WheelSurfaceSpeed : Outport  Port=3
  TorqueAvailable : Outport  Port=4
  TorqueCommand : Outport  Port=5
  wires:
  WheelRadius/1 -> WheelSurfaceSpeed/1
  ElectricalPower/1 -> MotorPower/1
  MotorMechanicalPower/1 -> ElectricalPower/1
  WheelInertia/1 -> WheelOmega/1
  WheelTorqueBalance/1 -> WheelInertia/1
  TireTorque/1 -> WheelTorqueBalance/2
  TireForce/1 -> TireTorque/1
  FinalDrive/1 -> WheelTorqueBalance/1
  MotorBandwidth/1 -> MotorTorqueState/1
  MotorTorqueError/1 -> MotorBandwidth/1
  MotorTorqueState/1 -> FinalDrive/1, MotorTorque/1, MotorTorqueError/2
  ApplyPowerScale/1 -> MotorTorqueError/1, TorqueCommand/1
  ApplySpeedLimit/1 -> ApplyPowerScale/1, MotorMechanicalPower/1
  AvailableAtSpeed/1 -> TorqueAvailable/1
  AvailableTorque/1 -> AvailableAtSpeed/1
  PowerScale/1 -> ApplyPowerScale/2, AvailableTorque/1
  WheelOmega/1 -> MotorMechanicalPower/2, WheelRadius/1, SpeedMargin/2
  TorqueRequested/1 -> ApplySpeedLimit/1
  MaxWheelOmega/1 -> SpeedMargin/1
  SpeedMargin/1 -> TaperGain/1
  TaperGain/1 -> SpeedLimitTaper/1
  SpeedLimitTaper/1 -> ApplySpeedLimit/2, AvailableAtSpeed/2

== system TC_track/Wheel_FL/Slip_Estimator ==
  VehicleSpeed : Inport
  WheelSurfaceSpeed : Inport  Port=2
  SlipDenominator : MinMax  Function=max  Inputs=2
  SlipNumerator : Sum  Inputs=+-
  SlipRatio : Product  Inputs=*/
  SlipSpeedFloor : Constant  Value=slipSpeedFloor
  Slip : Outport
  wires:
  SlipRatio/1 -> Slip/1
  SlipDenominator/1 -> SlipRatio/2
  SlipNumerator/1 -> SlipRatio/1
  SlipSpeedFloor/1 -> SlipDenominator/2
  VehicleSpeed/1 -> SlipDenominator/1, SlipNumerator/2
  WheelSurfaceSpeed/1 -> SlipNumerator/1

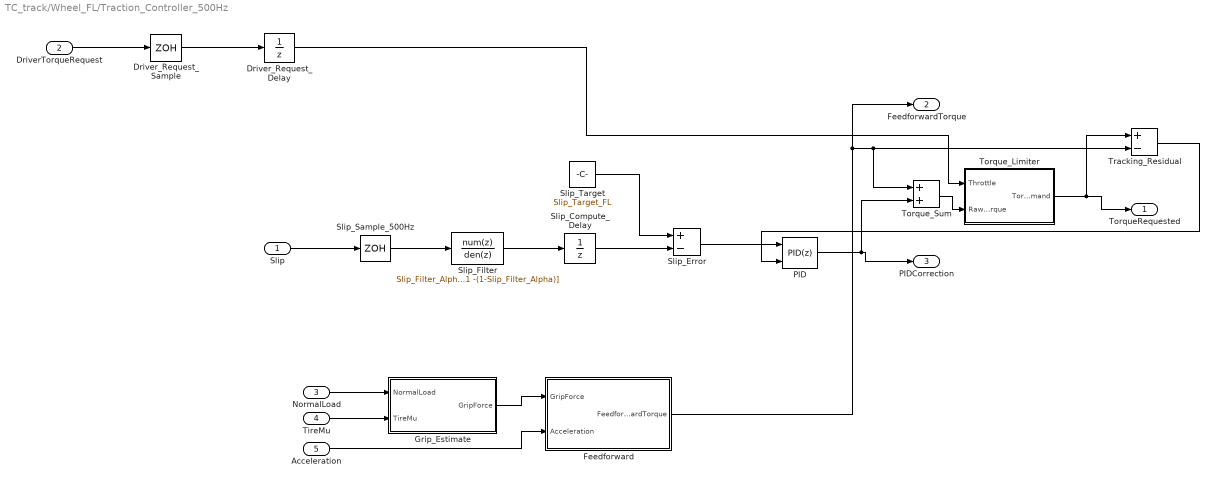
== system TC_track/Wheel_FL/Traction_Controller_500Hz ==
  Slip : Inport
  DriverTorqueRequest : Inport  Port=2
  NormalLoad : Inport  Port=3
  TireMu : Inport  Port=4
  Acceleration : Inport  Port=5
  Driver_Request_Delay : UnitDelay  InitialCondition=Launch_Pedal_Initial  SampleTime=Ts
  Driver_Request_Sample : ZeroOrderHold  SampleTime=Ts
  Feedforward : Subsystem
  Grip_Estimate : Subsystem
  PID : slpidlib/PID Controller  Controller=PID  Form=Parallel  TimeDomain=Discrete-time  UseExternalTs=off  SampleTime=Ts  IntegratorMethod=Forward Euler  FilterMethod=Forward Euler  ControllerParametersSource=internal  P=Kp_FL  I=Ki_FL  UseKiTs=off  D=Kd_FL  UseExternalDerivativeSource=off  N=100  UseFilter=on  TunerSelectOption=Transfer Function Based (PID Tuner App)  InitialConditionSource=internal  InitialConditionForIntegrator=0  InitialConditionForFilter=0  DifferentiatorICPrevScaledInput=0  ExternalReset=none  TrackingMode=on  Kt=Ktrack_FL  LimitOutput=on  SatLimitsSource=internal  UpperSaturationLimit=Cmax  LowerSaturationLimit=Cmin  LinearizeAsGain=on  AntiWindupMode=back-calculation  Kb=Kaw_FL  LimitIntegrator=off  UpperIntegratorSaturationLimit=inf  LowerIntegratorSaturationLimit=-inf  POutMin=[]  POutMax=[]  IOutMin=[]  IOutMax=[]  DOutMin=[]  DOutMax=[]  NOutMin=[]  NOutMax=[]  SumOutMin=[]  SumOutMax=[]  SaturationOutMin=[]  SaturationOutMax=[]  PParamMin=[]  PParamMax=[]  IParamMin=[]  IParamMax=[]  DParamMin=[]  DParamMax=[]  NParamMin=[]  NParamMax=[]  KbParamMin=[]  KbParamMax=[]  KtParamMin=[]  KtParamMax=[]  KbOutMin=[]  KbOutMax=[]  KtOutMin=[]  KtOutMax=[]  IntegratorOutMin=[]  IntegratorOutMax=[]  FilterOutMin=[]  FilterOutMax=[]  SumI1OutMin=[]  SumI1OutMax=[]  SumI2OutMin=[]  SumI2OutMax=[]  SumI3OutMin=[]  SumI3OutMax=[]  SumI4OutMin=[]  SumI4OutMax=[]  SumDOutMin=[]  SumDOutMax=[]  DifferentiatorOutMin=[]  DifferentiatorOutMax=[]  FilterDiffOutCoefMin=[]  FilterDiffOutCoefMax=[]  ReciprocalOutMin=[]  ReciprocalOutMax=[]  SumDenOutMin=[]  SumDenOutMax=[]  SumNumOutMin=[]  SumNumOutMax=[]  DivideOutMin=[]  DivideOutMax=[]  UdiffTsProdOutMin=[]  UdiffTsProdOutMax=[]  NTsProdOutMin=[]  NTsProdOutMax=[]  UintegralTsProdOutMin=[]  UintegralTsProdOutMax=[]  UngainTsProdOutMin=[]  UngainTsProdOutMax=[]  ClampingZeroOutDataTypeStr=Inherit: Inherit via back propagation  ClampingZeroOutMin=[]  ClampingZeroOutMax=[]  FilterDenConstantOutDataTypeStr=Inherit: Inherit via back propagation  FilterDenConstantOutMin=[]  FilterDenConstantOutMax=[]  PCopyOutDataTypeStr=Inherit: Inherit via back propagation  PCopyOutMin=[]  PCopyOutMax=[]  NCopyOutDataTypeStr=Inherit: Inherit via back propagation  NCopyOutMin=[]  NCopyOutMax=[]  IntegratorContinuousStateAttributes=''  IntegratorStateMustResolveToSignalObject=off  IntegratorRTWStateStorageClass=Auto  FilterContinuousStateAttributes=''  FilterStateMustResolveToSignalObject=off  FilterRTWStateStorageClass=Auto  ParallelPVariant=InternalParameters  IdealPVariant=Disabled  IVariant=InternalParameters  DVariant=InternalParameters  IntegratorVariant=Discrete  SatVariant=Enabled  AWVariant=BackCalculation  PCopyVariant=Disabled  TRVariant=Enabled  FdbkBlocksVariant=Forward  IdealPFdbkVariant=Disabled  SatFdbkVariant=Disabled  DerivativeFilterVariant=ForwardEulerFilter  NVariant=InternalParameters  NCopyVariant=Disabled  FilterICVariant=InternalICsFilter  IntegratorICVariant=InternalICs  ExternalResetVariant=Disabled  TRSumVariant=TrackingMode  SumFdbkVariant=Disabled  SumVariant=Sum_PID  TsampFilterVariant=InternalTs  TsampNgainVariant=Passthrough  TsampIntegralVariant=Disabled_SignalSpec  ExternalSaturationOutDataTypeStr=Inherit: Same as second input  DerivativeSourceVariant=ErrorSignal  PreIntVariant=InternalPreInt
  Slip_Compute_Delay : UnitDelay  SampleTime=Ts
  Slip_Error : Sum  Inputs=+-
  Slip_Filter : DiscreteFilter  Numerator=Slip_Filter_Alpha  Denominator=[1 -(1-Slip_Filter_Alpha)]  SampleTime=Ts
  Slip_Sample_500Hz : ZeroOrderHold  SampleTime=Ts
  Slip_Target : Constant  Value=Slip_Target_FL
  Torque_Limiter : Subsystem
  Torque_Sum : Sum
  Tracking_Residual : Sum  Inputs=+-
  TorqueRequested : Outport
  FeedforwardTorque : Outport  Port=2
  PIDCorrection : Outport  Port=3
  wires:
  Tracking_Residual/1 -> PID/2
  PID/1 -> Torque_Sum/2, PIDCorrection/1
  Driver_Request_Sample/1 -> Driver_Request_Delay/1
  DriverTorqueRequest/1 -> Driver_Request_Sample/1
  Slip_Error/1 -> PID/1
  Slip_Compute_Delay/1 -> Slip_Error/2
  Slip_Target/1 -> Slip_Error/1
  Slip_Filter/1 -> Slip_Compute_Delay/1
  Slip_Sample_500Hz/1 -> Slip_Filter/1
  Slip/1 -> Slip_Sample_500Hz/1
  Feedforward/1(FeedforwardTorque) -> Torque_Sum/1, Tracking_Residual/2, FeedforwardTorque/1
  NormalLoad/1 -> Grip_Estimate/1(NormalLoad)
  TireMu/1 -> Grip_Estimate/2(TireMu)
  Grip_Estimate/1(GripForce) -> Feedforward/1(GripForce)
  Acceleration/1 -> Feedforward/2(Acceleration)
  Torque_Limiter/1(TorqueCommand) -> TorqueRequested/1, Tracking_Residual/1
  Driver_Request_Delay/1 -> Torque_Limiter/1(Throttle)
  Torque_Sum/1 -> Torque_Limiter/2(RawTorque)

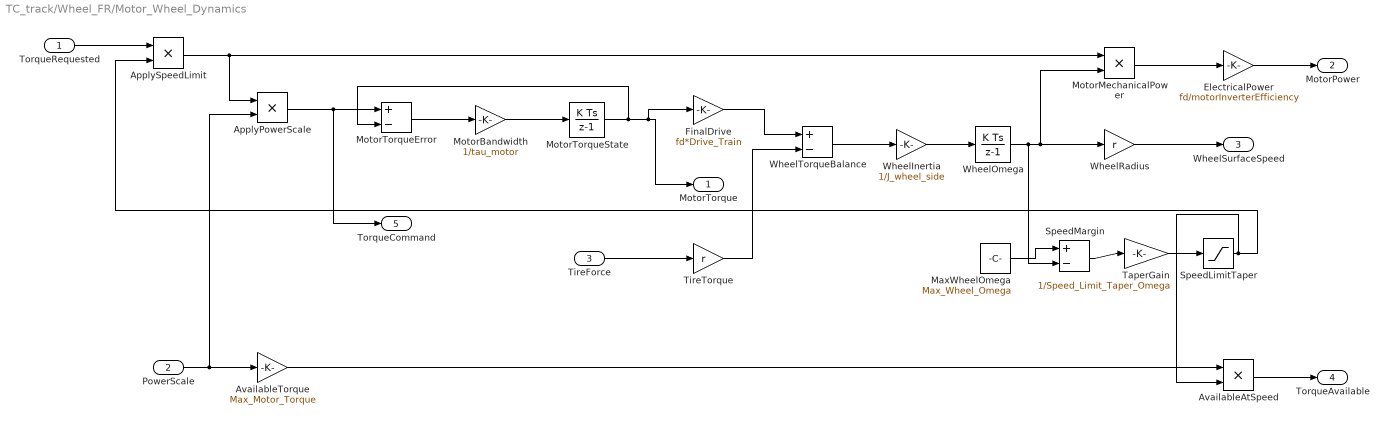
== system TC_track/Wheel_FR/Motor_Wheel_Dynamics ==
  TorqueRequested : Inport
  PowerScale : Inport  Port=2
  TireForce : Inport  Port=3
  ApplyPowerScale : Product  Inputs=**
  ApplySpeedLimit : Product  Inputs=**
  AvailableAtSpeed : Product  Inputs=**
  AvailableTorque : Gain  Gain=Max_Motor_Torque
  ElectricalPower : Gain  Gain=fd/motorInverterEfficiency
  FinalDrive : Gain  Gain=fd*Drive_Train
  MaxWheelOmega : Constant  Value=Max_Wheel_Omega
  MotorBandwidth : Gain  Gain=1/tau_motor
  MotorMechanicalPower : Product  Inputs=**
  MotorTorqueError : Sum  Inputs=+-
  MotorTorqueState : DiscreteIntegrator  SampleTime=Ts_plant  ICPrevOutput=DiscIntNeverNeededParam  ICPrevScaledInput=DiscIntNeverNeededParam
  SpeedLimitTaper : Saturate  UpperLimit=1  LowerLimit=0
  SpeedMargin : Sum  Inputs=+-
  TaperGain : Gain  Gain=1/Speed_Limit_Taper_Omega
  TireTorque : Gain  Gain=r
  WheelInertia : Gain  Gain=1/J_wheel_side
  WheelOmega : DiscreteIntegrator  SampleTime=Ts_plant  ICPrevOutput=DiscIntNeverNeededParam  ICPrevScaledInput=DiscIntNeverNeededParam
  WheelRadius : Gain  Gain=r
  WheelTorqueBalance : Sum  Inputs=+-
  MotorTorque : Outport
  MotorPower : Outport  Port=2
  WheelSurfaceSpeed : Outport  Port=3
  TorqueAvailable : Outport  Port=4
  TorqueCommand : Outport  Port=5
  wires:
  AvailableAtSpeed/1 -> TorqueAvailable/1
  WheelRadius/1 -> WheelSurfaceSpeed/1
  ElectricalPower/1 -> MotorPower/1
  MotorMechanicalPower/1 -> ElectricalPower/1
  WheelInertia/1 -> WheelOmega/1
  WheelTorqueBalance/1 -> WheelInertia/1
  TireTorque/1 -> WheelTorqueBalance/2
  FinalDrive/1 -> WheelTorqueBalance/1
  TireForce/1 -> TireTorque/1
  MotorBandwidth/1 -> MotorTorqueState/1
  MotorTorqueError/1 -> MotorBandwidth/1
  MotorTorqueState/1 -> FinalDrive/1, MotorTorque/1, MotorTorqueError/2
  ApplyPowerScale/1 -> MotorTorqueError/1, TorqueCommand/1
  ApplySpeedLimit/1 -> ApplyPowerScale/1, MotorMechanicalPower/1
  AvailableTorque/1 -> AvailableAtSpeed/1
  PowerScale/1 -> ApplyPowerScale/2, AvailableTorque/1
  WheelOmega/1 -> MotorMechanicalPower/2, WheelRadius/1, SpeedMargin/2
  TorqueRequested/1 -> ApplySpeedLimit/1
  MaxWheelOmega/1 -> SpeedMargin/1
  SpeedMargin/1 -> TaperGain/1
  TaperGain/1 -> SpeedLimitTaper/1
  SpeedLimitTaper/1 -> ApplySpeedLimit/2, AvailableAtSpeed/2

== system TC_track/Wheel_FR/Slip_Estimator ==
  VehicleSpeed : Inport
  WheelSurfaceSpeed : Inport  Port=2
  SlipDenominator : MinMax  Function=max  Inputs=2
  SlipNumerator : Sum  Inputs=+-
  SlipRatio : Product  Inputs=*/
  SlipSpeedFloor : Constant  Value=slipSpeedFloor
  Slip : Outport
  wires:
  SlipRatio/1 -> Slip/1
  SlipDenominator/1 -> SlipRatio/2
  SlipNumerator/1 -> SlipRatio/1
  SlipSpeedFloor/1 -> SlipDenominator/2
  VehicleSpeed/1 -> SlipDenominator/1, SlipNumerator/2
  WheelSurfaceSpeed/1 -> SlipNumerator/1
